simulink model "test_NO_OBSERVER_sweep"  (R2020a)
settings: Solver=ode15s  StartTime=0.0  StopTime=100  FixedStep=1/fs  MaxStep=1/(2*fs)  RelTol=1e-6
undefined symbols (not defined in the file): A, A_reduc, Amp, B, B_reduc, Bdlol, C_reduc, Cc, D, den_anti, den_mems, DiscIntNeverNeededParam, f0, fs, g, L, Li, Lobs, n_adc, NSD_mems, num_anti, num_mems, obs_i_den, obs_i_num, obs_x2_den, obs_x2_num, R, sens_mems, v0, Vcc, Vmax_ADC, Vmin_ADC, x0
libraries: simulink x2, dspstat3 x1, simulink_extras x1
settings Model: Creator=Noxi-PC  LastModifiedBy=Noxi-PC
settings SolverCC: ZeroCrossAlgorithm=Adaptive  AlgebraicLoopSolver=LineSearch
settings DebuggingCC: IgnoredZcDiagnostic=none

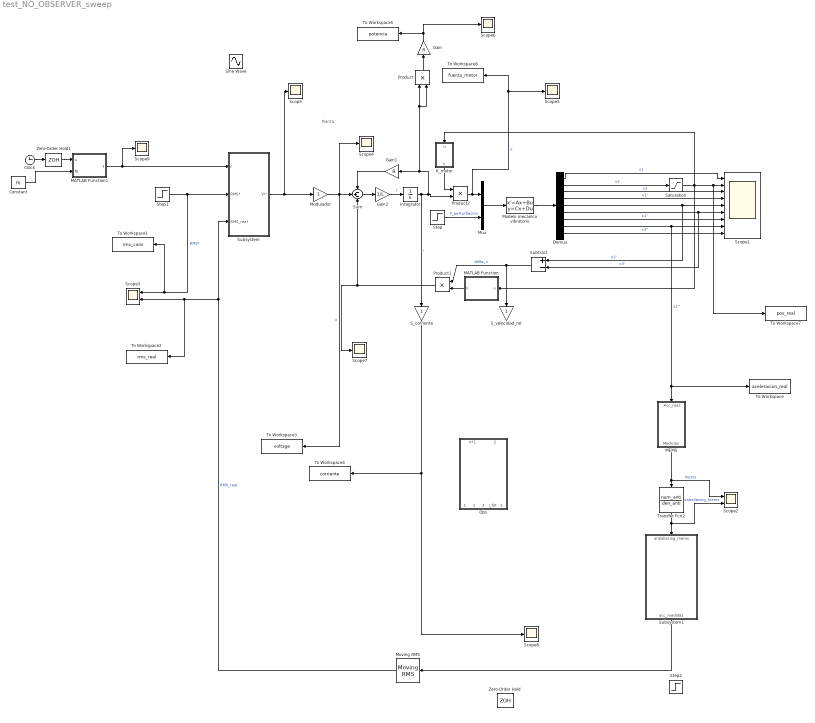
== system test_NO_OBSERVER_sweep ==
  note: Planta
  Clock : Clock
  Constant : Constant  Value=f0
  Demux : Demux  Outputs=9
  Gain : Gain  Gain=R
  Gain1 : Gain  Gain=R
  Gain2 : Gain  Gain=1/L
  Integrator : Integrator
  K_motor : MATLAB Function  TreatAsAtomicUnit=on
  MATLAB Function : MATLAB Function  TreatAsAtomicUnit=on
  MATLAB Function1 : MATLAB Function  TreatAsAtomicUnit=on
  MEMS : Subsystem
  Modelo mecánico vibratorio : StateSpace  A=A  B=B  C=Cc  D=D  InitialCondition=[x0,v0]
  Modulador : Gain
  Moving RMS : dspstat3/Moving RMS  Method=Sliding window  ForgettingFactorPort=off  SpecifyWindowLength=on  WindowLength=Ventana  ForgettingFactor=0.99  SimulateUsing=Interpreted execution
      settings: SourceProductBaseCode=DS
  Mux : Mux  Inputs=2
  Obs : Subsystem
  Product : Product
  Product1 : Product
  Product2 : Product
  S_corriente : Gain
  S_velocidad_rel : Gain
  Saturation : Saturate  UpperLimit=12.7e-3  LowerLimit=-12.7e-3
  Scope{,4..7,9} (6 alike) : Scope
  Scope1 : Scope  NumInputPorts=9
  Scope2 : Scope  NumInputPorts=2
  Scope3 : Scope  NumInputPorts=2
  Scope8 : Scope  NumInputPorts=3
  Sine Wave : Sin  Amplitude=5  Frequency=2*pi*f0  SampleTime=0
  Step : Step  After=0  SampleTime=0
  Step1 : Step  Time=0  After=Amp/sqrt(2)  SampleTime=0
  Step2 : Step  SampleTime=0
  Subsystem : Subsystem
  Subsystem1 : Subsystem
  Subtract : Sum  Inputs=+-
  Sum : Sum  Inputs=-+-
  To Workspace : ToWorkspace  VariableName=aceleracion_real  SaveFormat=Structure With Time  SampleTime=-1
  To Workspace1 : ToWorkspace  VariableName=rms_cons  SaveFormat=Structure With Time  SampleTime=-1
  To Workspace2 : ToWorkspace  VariableName=rms_real  SaveFormat=Structure With Time  SampleTime=-1
  To Workspace3 : ToWorkspace  VariableName=voltage  SaveFormat=Structure With Time  SampleTime=-1
  To Workspace4 : ToWorkspace  VariableName=corriente  SaveFormat=Structure With Time  SampleTime=-1
  To Workspace5 : ToWorkspace  VariableName=potencia  SaveFormat=Structure With Time  SampleTime=-1
  To Workspace6 : ToWorkspace  VariableName=fuerza_motor  SaveFormat=Structure With Time  SampleTime=-1
  To Workspace7 : ToWorkspace  VariableName=pos_real  SaveFormat=Structure With Time  SampleTime=-1
  Transfer Fcn2 : TransferFcn  Numerator=num_anti  Denominator=den_anti
  Zero-Order Hold : ZeroOrderHold  SampleTime=1/fs
  Zero-Order Hold1 : ZeroOrderHold  SampleTime=1/fs
  wires:
  Modelo mecánico vibratorio/1 -> Demux/1
  Demux/1 -> Scope1/1  "x1"
  Demux/2 -> Saturation/1  "x2"
  Demux/3 -> Scope1/3  "x3"
  Demux/4 -> Scope1/4  "x1'"
  Demux/5 -> Scope1/5, Subtract/1  "x2'"
  Demux/6 -> Scope1/6, Subtract/2  "x3'"
  Demux/7 -> Scope1/7  "x1''"
  Demux/8 -> MEMS/1(Acc_real), To Workspace/1, Scope1/8  "x2''"
  Demux/9 -> Scope1/9  "x3''"
  Mux/1 -> Modelo mecánico vibratorio/1
  Sum/1 -> Gain2/1
  Integrator/1 -> S_corriente/1, Product2/2, Gain1/1, Product/2, Product/1  "i"
  Gain1/1 -> Sum/1
  Gain2/1 -> Integrator/1  "i'"
  Step/1 -> Mux/2  "F_perturbación"
  Product1/1 -> Scope7/1, Sum/3
  Subtract/1 -> Product1/1, S_velocidad_rel/1  "delta_v"
  Modulador/1 -> Scope4/1, To Workspace3/1, Sum/2  "V"
  Saturation/1 -> K_motor/1(u), MATLAB Function/1(u), To Workspace7/1, Scope1/2
  Product2/1 -> To Workspace6/1, Scope5/1, Mux/1  "F"
  K_motor/1(k) -> Product2/1
  MATLAB Function/1(k) -> Product1/2
  MATLAB Function1/1(f) -> Subsystem/1(f), Scope9/1
  Step1/1 -> Scope3/1, To Workspace1/1, Subsystem/2(RMS*)  "RMS*"
  Subsystem/1(V*') -> Scope/1, Modulador/1
  MEMS/1(Medición) -> Scope2/1, Transfer Fcn2/1  "mems"
  Moving RMS/1 -> Subsystem/3(RMS_real), To Workspace2/1, Scope3/2  "RMS_real"
  Transfer Fcn2/1 -> Scope2/2, Subsystem1/1(antialiasing_mems)  "antialiasing_mems"
  S_corriente/1 -> To Workspace4/1, Scope8/2
  Subsystem1/1(acc_medida1) -> Moving RMS/1
  Product/1 -> Gain/1
  Gain/1 -> To Workspace5/1, Scope6/1
  Zero-Order Hold1/1 -> MATLAB Function1/1(u)
  Constant/1 -> MATLAB Function1/2(f0)
  Clock/1 -> Zero-Order Hold1/1

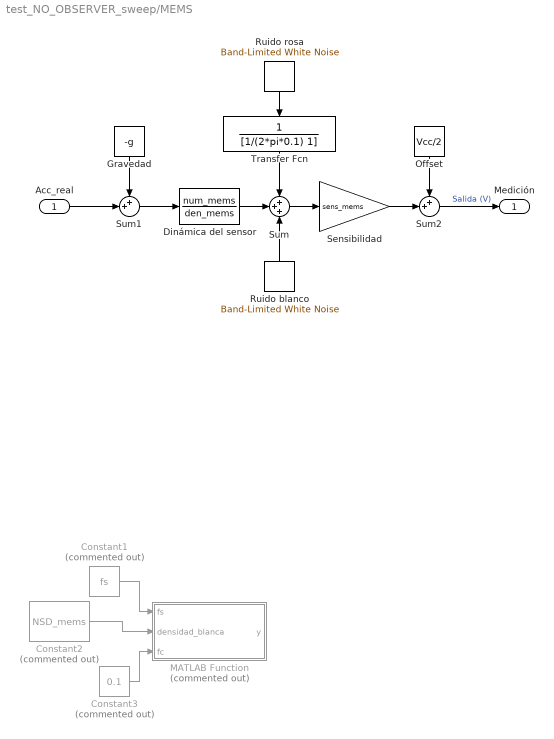
== system test_NO_OBSERVER_sweep/MEMS ==
  Acc_real : Inport
  Constant1 : Constant  Commented=on  Value=fs
  Constant2 : Constant  Commented=on  Value=NSD_mems
  Constant3 : Constant  Commented=on  Value=0.1
  Dinámica del sensor : TransferFcn  Numerator=num_mems  Denominator=den_mems
  Gravedad : Constant  Value=-g
  MATLAB Function : MATLAB Function  Commented=on  TreatAsAtomicUnit=on
  Offset : Constant  Value=Vcc/2
  Ruido blanco : simulink/Sources/Band-Limited White Noise  Cov=PSD_mems  Ts=1/3*1/fs  seed=[2674]
  Ruido rosa : simulink/Sources/Band-Limited White Noise  Cov=PSD_mems  Ts=1/3*1/fs  seed=[26744]
  Sensibilidad : Gain  Gain=sens_mems
  Sum : Sum  Inputs=+++
  Sum1 : Sum  Inputs=++|
  Sum2 : Sum  Inputs=++|
  Transfer Fcn : TransferFcn  Denominator=[1/(2*pi*0.1) 1]
  Medición : Outport
  wires:
  Sum1/1 -> Dinámica del sensor/1
  Acc_real/1 -> Sum1/2
  Sum/1 -> Sensibilidad/1
  Sensibilidad/1 -> Sum2/2
  Sum2/1 -> Medición/1  "Salida (V)"
  Gravedad/1 -> Sum1/1
  Offset/1 -> Sum2/1
  Constant1/1 -> MATLAB Function/1(fs)
  Constant2/1 -> MATLAB Function/2(densidad_blanca)
  Constant3/1 -> MATLAB Function/3(fc)
  Ruido blanco/1 -> Sum/3
  Ruido rosa/1 -> Transfer Fcn/1
  Dinámica del sensor/1 -> Sum/2
  Transfer Fcn/1 -> Sum/1

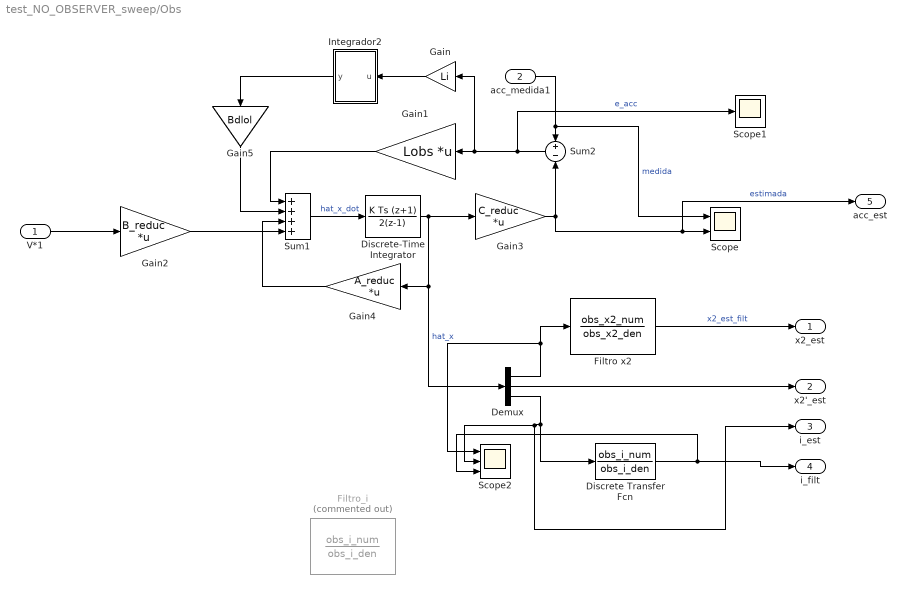
== system test_NO_OBSERVER_sweep/Obs ==
  V*1 : Inport
  acc_medida1 : Inport  Port=2
  Demux : Demux  Outputs=3
  Discrete Transfer Fcn : DiscreteTransferFcn  Numerator=obs_i_num  Denominator=obs_i_den  SampleTime=1/fs
  Discrete-Time Integrator : DiscreteIntegrator  IntegratorMethod=Integration: Trapezoidal  SampleTime=1/fs  ICPrevOutput=DiscIntNeverNeededParam  ICPrevScaledInput=DiscIntNeverNeededParam
  Filtro x2 : TransferFcn  Numerator=obs_x2_num  Denominator=obs_x2_den
  Filtro_i : TransferFcn  Commented=on  Numerator=obs_i_num  Denominator=obs_i_den
  Gain : Gain  Gain=Li
  Gain1 : Gain  Gain=Lobs  Multiplication=Matrix(K*u)
  Gain2 : Gain  Gain=B_reduc  Multiplication=Matrix(K*u)
  Gain3 : Gain  Gain=C_reduc  Multiplication=Matrix(K*u)
  Gain4 : Gain  Gain=A_reduc  Multiplication=Matrix(K*u)
  Gain5 : Gain  Gain=Bdlol
  Integrador2 : Subsystem
  Scope : Scope  NumInputPorts=2
  Scope1 : Scope
  Scope2 : Scope  NumInputPorts=3
  Sum1 : Sum  Inputs=++++
  Sum2 : Sum  Inputs=+|-
  x2_est : Outport
  x2'_est : Outport  Port=2
  i_est : Outport  Port=3
  i_filt : Outport  Port=4
  acc_est : Outport  Port=5
  wires:
  Gain1/1 -> Sum1/1
  Gain4/1 -> Sum1/3
  V*1/1 -> Gain2/1
  Sum2/1 -> Scope1/1, Gain/1, Gain1/1  "e_acc"
  Discrete-Time Integrator/1 -> Demux/1, Gain4/1, Gain3/1  "hat_x"
  Sum1/1 -> Discrete-Time Integrator/1  "hat_x_dot"
  acc_medida1/1 -> Scope/1, Sum2/1  "medida"
  Gain3/1 -> Sum2/2, acc_est/1, Scope/2  "estimada"
  Gain/1 -> Integrador2/1(u)
  Integrador2/1(y) -> Gain5/1
  Gain2/1 -> Sum1/4
  Demux/1 -> Scope2/1, Filtro x2/1
  Filtro x2/1 -> x2_est/1  "x2_est_filt"
  Demux/2 -> x2'_est/1
  Demux/3 -> Discrete Transfer Fcn/1, i_est/1, Scope2/2
  Discrete Transfer Fcn/1 -> Scope2/3, i_filt/1
  Gain5/1 -> Sum1/2

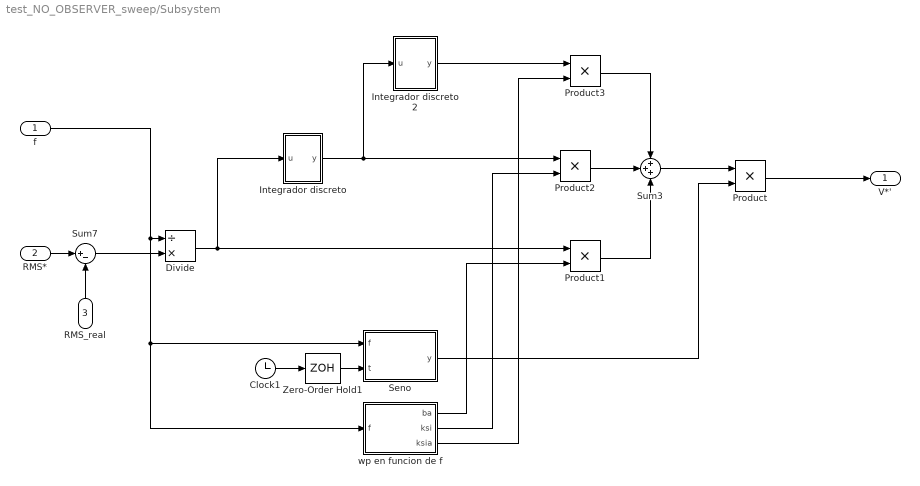
== system test_NO_OBSERVER_sweep/Subsystem ==
  f : Inport
  RMS* : Inport  Port=2
  RMS_real : Inport  Port=3
  Clock1 : Clock
  Divide : Product  Inputs=/*
  Integrador discreto : Subsystem
  Integrador discreto 2 : Subsystem
  Product{,1..3} (4 alike) : Product
  Seno : MATLAB Function  TreatAsAtomicUnit=on
  Sum3 : Sum  Inputs=+++
  Sum7 : Sum  Inputs=|+-
  Zero-Order Hold1 : ZeroOrderHold  SampleTime=1/fs
  wp en funcion de f : MATLAB Function  TreatAsAtomicUnit=on
  V*' : Outport
  wires:
  Integrador discreto 2/1(y) -> Product3/1
  Integrador discreto/1(y) -> Product2/1, Integrador discreto 2/1(u)
  RMS_real/1 -> Sum7/2
  RMS*/1 -> Sum7/1
  Product2/1 -> Sum3/2
  f/1 -> wp en funcion de f/1(f), Seno/1(f), Divide/1
  Sum3/1 -> Product/1
  Sum7/1 -> Divide/2
  Divide/1 -> Product1/1, Integrador discreto/1(u)
  Seno/1(y) -> Product/2
  Clock1/1 -> Zero-Order Hold1/1
  Zero-Order Hold1/1 -> Seno/2(t)
  Product3/1 -> Sum3/1
  Product1/1 -> Sum3/3
  Product/1 -> V*'/1
  wp en funcion de f/1(ba) -> Product1/2
  wp en funcion de f/2(ksi) -> Product2/2
  wp en funcion de f/3(ksia) -> Product3/2

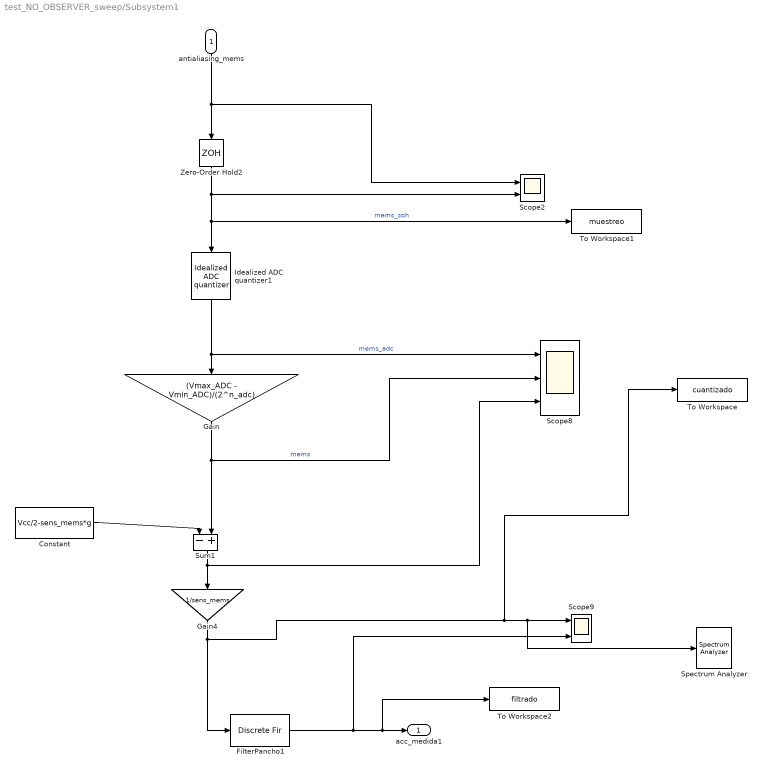
== system test_NO_OBSERVER_sweep/Subsystem1 ==
  antialiasing_mems : Inport
  Constant : Constant  Value=Vcc/2-sens_mems*g
  FilterPancho1 : DiscreteFir  Tag=BlockMethodSubSystem  Coefficients=[0 0.00944240077011487475 0.0474851918474631096 0.121195470415369752 0.202517996471183348 0.23871788099173788 0.202517996471183348 0.121195470415369752 0.0474851918474631096 0.00944240077011487475 0]  InputProcessing=Columns as channels (frame based)
  Gain : Gain  Gain=(Vmax_ADC - Vmin_ADC)/(2^n_adc)
  Gain4 : Gain  Gain=1/sens_mems
  Idealized ADC quantizer1 : simulink_extras/Additional Discrete/Idealized ADC quantizer  NumberOfConverterBits=n_adc  Vmin=Vmin_ADC  Vmax=Vmax_ADC  OutputDataType=uint16  OutputNegativeValues=off
  Scope2 : Scope  NumInputPorts=2
  Scope8 : Scope  NumInputPorts=3
  Scope9 : Scope  NumInputPorts=2
  Spectrum Analyzer : SpectrumAnalyzer
  Sum1 : Sum  Inputs=-+
  To Workspace : ToWorkspace  VariableName=cuantizado  SaveFormat=Structure With Time  SampleTime=1/fs
  To Workspace1 : ToWorkspace  VariableName=muestreo  SaveFormat=Structure With Time  SampleTime=1/fs
  To Workspace2 : ToWorkspace  VariableName=filtrado  SaveFormat=Structure With Time  SampleTime=1/fs
  Zero-Order Hold2 : ZeroOrderHold  SampleTime=1/(fs)
  acc_medida1 : Outport
  wires:
  Gain4/1 -> FilterPancho1/1, To Workspace/1, Spectrum Analyzer/1, Scope9/1
  Gain/1 -> Scope8/2, Sum1/2  "mems"
  Idealized ADC quantizer1/1 -> Gain/1, Scope8/1  "mems_adc"
  Sum1/1 -> Scope8/3, Gain4/1
  antialiasing_mems/1 -> Scope2/1, Zero-Order Hold2/1
  Zero-Order Hold2/1 -> To Workspace1/1, Idealized ADC quantizer1/1, Scope2/2  "mems_zoh"
  FilterPancho1/1 -> Scope9/2, To Workspace2/1, acc_medida1/1
  Constant/1 -> Sum1/1

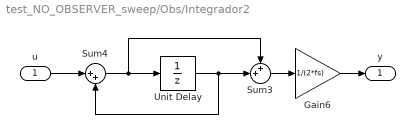
== system test_NO_OBSERVER_sweep/Obs/Integrador2 ==
  u : Inport
  Gain6 : Gain  Gain=1/(2*fs)
  Sum3 : Sum  Inputs=++|
  Sum4 : Sum  Inputs=|++
  Unit Delay : UnitDelay  SampleTime=1/fs  HasFrameUpgradeWarning=on
  y : Outport
  wires:
  Sum3/1 -> Gain6/1
  Sum4/1 -> Sum3/1, Unit Delay/1
  Unit Delay/1 -> Sum3/2, Sum4/2
  Gain6/1 -> y/1
  u/1 -> Sum4/1

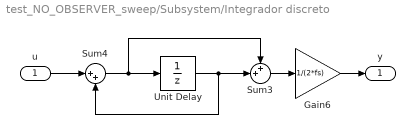
== system test_NO_OBSERVER_sweep/Subsystem/Integrador discreto ==
  u : Inport
  Gain6 : Gain  Gain=1/(2*fs)
  Sum3 : Sum  Inputs=++|
  Sum4 : Sum  Inputs=|++
  Unit Delay : UnitDelay  SampleTime=1/fs  HasFrameUpgradeWarning=on
  y : Outport
  wires:
  Sum3/1 -> Gain6/1
  Sum4/1 -> Sum3/1, Unit Delay/1
  Unit Delay/1 -> Sum3/2, Sum4/2
  Gain6/1 -> y/1
  u/1 -> Sum4/1

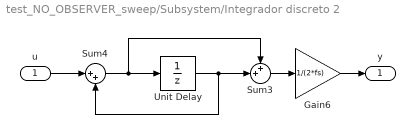
== system test_NO_OBSERVER_sweep/Subsystem/Integrador discreto 2 ==
  u : Inport
  Gain6 : Gain  Gain=1/(2*fs)
  Sum3 : Sum  Inputs=++|
  Sum4 : Sum  Inputs=|++
  Unit Delay : UnitDelay  SampleTime=1/fs  HasFrameUpgradeWarning=on
  y : Outport
  wires:
  Sum3/1 -> Gain6/1
  Sum4/1 -> Sum3/1, Unit Delay/1
  Unit Delay/1 -> Sum3/2, Sum4/2
  Gain6/1 -> y/1
  u/1 -> Sum4/1

== matlab function test_NO_OBSERVER_sweep/K_motor ==
  data: u input; k output
function k = fcn(u)
coefs = [1.88388325014986e-06,1.21220914940963e-07,-0.000604988778285308,-0.000369001905871298,-0.0433714523559467,-0.0474444922489168,51.4222931299995];

k = coefs(1)*u^6+coefs(2)*u^5+coefs(3)*u^4+coefs(4)*u^3+coefs(5)*u^2+coefs(6)*u^1+coefs(7);

== matlab function test_NO_OBSERVER_sweep/MATLAB Function ==
  data: u input; k output
function k= fcn(u)
coefs = [1883883250149.81,121220914.941173,-604988778.285297,-369001.905871325,-43371.4523559472,-47.4444922489166,51.4222931299995];

k = coefs(1)*u^6+coefs(2)*u^5+coefs(3)*u^4+coefs(4)*u^3+coefs(5)*u^2+coefs(6)*u^1+coefs(7);

== matlab function test_NO_OBSERVER_sweep/MEMS/MATLAB Function ==
  data: fs input; y output; densidad_blanca input; fc input
function y = ruido_sensor(fs, densidad_blanca, fc)

% Persistent state
persistent b a z

if isempty(b)
    [b, a] = butter(1, fc/(fs/2));
    z = 0;  % Estado inicial del filtro
end

% Ruido blanco
ruido_blanco = densidad_blanca * randn * sqrt(fs);

% Ruido 1/f (drift)
[ruido_drift, z] = filter(b, a, randn, z);

% Señal total
y = ruido_blanco + ruido_drift;

== matlab function test_NO_OBSERVER_sweep/Subsystem/Seno ==
  data: f input; y output; t input
function y = fcn(f,t)

y = sin(2*pi*f*t);

== matlab function test_NO_OBSERVER_sweep/MATLAB Function1 ==
  data: u input; f output; f0 input
function f = fcn(u,f0)

f = f0* 2^(2*u/60);

== matlab function test_NO_OBSERVER_sweep/Subsystem/wp en funcion de f ==
  data: f input; ba output; ksi output; ksia output
function [ba,ksi,ksia] = fcn(f)
m_movil = 0.94;
zita = 0.7;
wp = wpfreq(f);
R_control = 9.5;
K_motor = 51.6;
ba = m_movil*(2*zita+1)*wp*R_control/(K_motor*2*pi*f);
ksi = m_movil*(2*zita+1)*wp^2*10*R_control/(K_motor*2*pi*f);
ksia = m_movil*wp^3*R_control/(K_motor*2*pi*f);
end

function wp = wpfreq(f)
    % Tabla de frecuencia (Hz) y valores correspondientes de wp
    freq_table = [ ...
          5,  10,  20,  25,  30,  40,  50,  60,  70,  80, ...
         90, 100, 200, 300, 400, 500, 600,700,800, 900, 1000, 1100,1200, 1300, 1450, 1500,1800, 2000];

    wp_table = [ ...
         20,  10,  15,  15,  15,  15,  15,  18,  20,  20, ...
         30,  20,  25,  30,  35, 35,40,60, 80, 80,  100, 100,100, 100, 100,  120,90,  100];

    % Interpolación lineal
    wp = interp1(freq_table, wp_table, f, 'linear', 'extrap');
end
